simulink model "TP801_control"  (R2018b)
settings: Solver=ode4  StartTime=0.0  StopTime=40  FixedStep=0.001  RelTol=1e-3  EnableMultiTasking=on
settings Model: Creator=ROBOTICA  LastModifiedBy=Daniel
settings DataIOCC: LimitDataPoints=on  SaveFormat=Array
settings OptimizationCC: LifeSpan=inf
settings DebuggingCC: UnderspecifiedInitializationDetection=Classic  MergeDetectMultiDrivingBlocksExec=none  SolverPrmCheckMsg=warning  AllowSymbolicDim=off  SFUnexpectedBacktrackingDiag=warning  SFNoUnconditionalDefaultTransitionDiag=warning  SFExecutionAtInitializationDiag=none
settings HardwareCC: ProdBitPerPointer=32  ProdBitPerSizeT=32  ProdBitPerPtrDiffT=32  ProdLargestAtomicFloat=None  ProdIntDivRoundTo=Undefined  ProdEndianess=Unspecified  ProdWordSize=32  ProdHWDeviceType=32-bit Generic
settings ModelReferenceCC: PropagateSignalLabelsOutOfModel=off
settings SFSimCC: SimUseLocalCustomCode=off
settings RTWCC: RTWUseLocalCustomCode=off
settings CodeAppCC: StateflowObjectComments=on
settings GRTTargetCC: TargetLangStandard=C89/C90 (ANSI)  GeneratePreprocessorConditionals=Disable all
settings ConfigComp: CovMetricSettings=dw  CovHtmlReporting=on  CovSaveCumulativeToWorkspaceVar=on  CovSaveSingleToWorkspaceVar=on  CovExternalEMLEnable=off

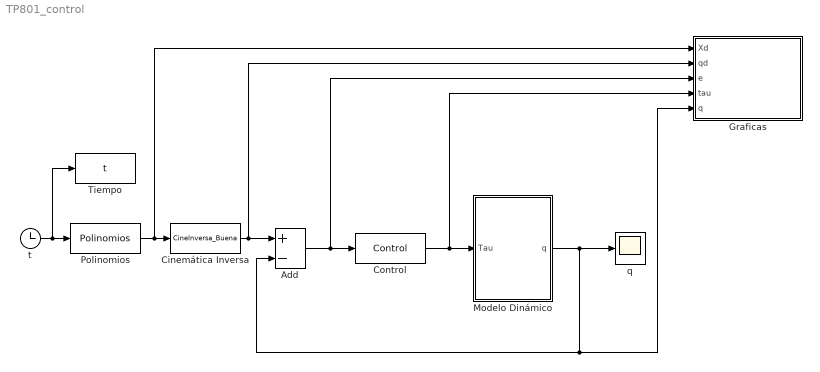
== system TP801_control ==
  " Cinemática Inversa" : MATLABFcn  MATLABFcn=CineInversa_Buena  OutputDimensions=3  Output1D=off
  Add : Sum  Inputs=+-
  Control : MATLABFcn  MATLABFcn=Control  OutputDimensions=3  Output1D=off
  Graficas : Subsystem
  Modelo Dinámico : Subsystem
  Polinomios : MATLABFcn  MATLABFcn=Polinomios  OutputDimensions=3  Output1D=off
  Tiempo : ToWorkspace  VariableName=t  SampleTime=-1
  q : Scope
  t : Clock
  wires:
  t/1 -> Tiempo/1, Polinomios/1
  Polinomios/1 -> Graficas/1(Xd), " Cinemática Inversa"/1
  " Cinemática Inversa"/1 -> Graficas/2(qd), Add/1
  Add/1 -> Graficas/3(e), Control/1
  Modelo Dinámico/1(q) -> Graficas/5(q), Add/2, q/1
  Control/1 -> Graficas/4(tau), Modelo Dinámico/1(Tau)

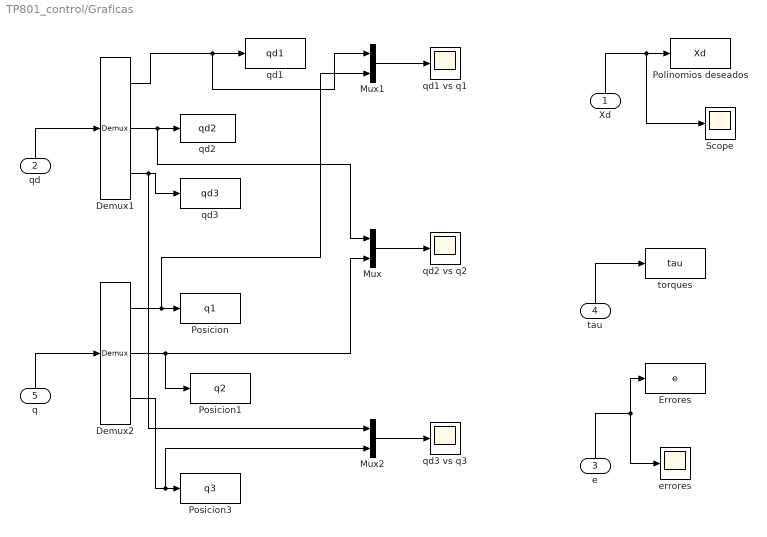
== system TP801_control/Graficas ==
  Xd : Inport
  qd : Inport  Port=2
  e : Inport  Port=3
  tau : Inport  Port=4
  q : Inport  Port=5
  Demux1 : Demux  Outputs=3
  Demux2 : Demux  Outputs=3
  Errores : ToWorkspace  VariableName=e  SampleTime=-1
  Mux : Mux  Inputs=2
  Mux1 : Mux  Inputs=2
  Mux2 : Mux  Inputs=2
  Polinomios deseados : ToWorkspace  VariableName=Xd  SampleTime=-1
  Posicion : ToWorkspace  VariableName=q1  SampleTime=-1
  Posicion1 : ToWorkspace  VariableName=q2  SampleTime=-1
  Posicion3 : ToWorkspace  VariableName=q3  SampleTime=-1
  Scope : Scope
  errores : Scope
  qd1 : ToWorkspace  VariableName=qd1  SampleTime=-1
  qd1 vs q1 : Scope
  qd2 : ToWorkspace  VariableName=qd2  SampleTime=-1
  qd2 vs q2 : Scope
  qd3 : ToWorkspace  VariableName=qd3  SampleTime=-1
  qd3 vs q3 : Scope
  torques : ToWorkspace  VariableName=tau  SampleTime=-1
  wires:
  e/1 -> errores/1, Errores/1
  tau/1 -> torques/1
  Xd/1 -> Scope/1, Polinomios deseados/1
  qd/1 -> Demux1/1
  Demux1/1 -> Mux1/1, qd1/1
  Demux1/2 -> Mux/1, qd2/1
  q/1 -> Demux2/1
  Demux2/3 -> Mux2/2, Posicion3/1
  Demux2/2 -> Mux/2, Posicion1/1
  Mux/1 -> qd2 vs q2/1
  Mux1/1 -> qd1 vs q1/1
  Demux2/1 -> Mux1/2, Posicion/1
  Mux2/1 -> qd3 vs q3/1
  Demux1/3 -> Mux2/1, qd3/1

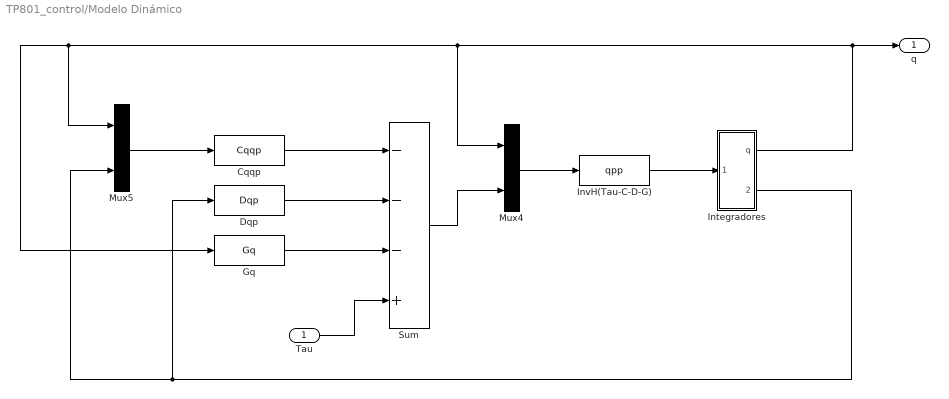
== system TP801_control/Modelo Dinámico ==
  Tau : Inport
  Cqqp : MATLABFcn  MATLABFcn=Cqqp  OutputDimensions=3  OutputSignalType=real
  Dqp : MATLABFcn  MATLABFcn=Dqp  OutputDimensions=3  OutputSignalType=real
  Gq : MATLABFcn  MATLABFcn=Gq  OutputDimensions=3  OutputSignalType=real
  Integradores : Subsystem
  InvH(Tau-C-D-G) : MATLABFcn  MATLABFcn=qpp  OutputDimensions=3  OutputSignalType=real
  Mux4 : Mux  Inputs=2
  Mux5 : Mux  Inputs=2
  Sum : Sum  Inputs=---+
  q : Outport
  wires:
  Tau/1 -> Sum/4
  Mux5/1 -> Cqqp/1
  Gq/1 -> Sum/3
  Cqqp/1 -> Sum/1
  Dqp/1 -> Sum/2
  Integradores/1(q) -> q/1, Mux4/1, Mux5/1, Gq/1
  Integradores/2(qp) -> Dqp/1, Mux5/2
  Sum/1 -> Mux4/2
  InvH(Tau-C-D-G)/1 -> Integradores/1(qpp)
  Mux4/1 -> InvH(Tau-C-D-G)/1

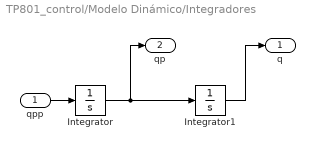
== system TP801_control/Modelo Dinámico/Integradores ==
  qpp : Inport
  Integrator : Integrator
  Integrator1 : Integrator  InitialCondition=[0 0.19 0.19]
  q : Outport
  qp : Outport  Port=2
  wires:
  Integrator/1 -> Integrator1/1, qp/1
  qpp/1 -> Integrator/1
  Integrator1/1 -> q/1
